simulink model "ScalarCalculator"  (R2021a)
settings: Solver=FixedStepDiscrete  StartTime=0.0  StopTime=10.0  RelTol=1e-3  EnableMultiTasking=on
libraries: simulink x2
settings Model: Creator=top one  LastModifiedBy=top one
settings DataIOCC: ReturnWorkspaceOutputs=off
settings OptimizationCC: DefaultParameterBehavior=Inlined  InlineInvariantSignals=on  EnableMemcpy=off  LifeSpan=1  EfficientTunableParamExpr=on
settings DebuggingCC: UnderspecifiedInitializationDetection=Classic  MergeDetectMultiDrivingBlocksExec=none  SFMachineParentedDataDiag=warning  ArithmeticOperatorsInVariantConditions=warning
settings ModelReferenceCC: PropagateSignalLabelsOutOfModel=off
settings SFSimCC: MATLABDynamicMemAlloc=off  CustomCodeUndefinedFunction=UseInterfaceOnly
settings RTWCC: SystemTargetFile=ert.tlc  GenCodeOnly=on  TemplateMakefile=ert_default_tmf  GenerateReport=on  IncludeHyperlinkInReport=on  LaunchReport=on  GenerateTraceInfo=on  GenerateTraceReport=on  GenerateTraceReportSl=on  GenerateTraceReportSf=on  GenerateTraceReportEml=on
settings CodeAppCC: ForceParamTrailComments=on  IgnoreCustomStorageClasses=off  OperatorAnnotations=on  SimulinkDataObjDesc=on  SFDataObjDesc=on  MATLABFcnDesc=on  InsertBlockDesc=on  StateflowObjectComments=on  MATLABSourceComments=on
settings ERTTargetCC: MultiwordLength=2048  GenerateSampleERTMain=on  InlinedParameterPlacement=NonHierarchical  ERTCustomFileTemplate=example_file_process.tlc

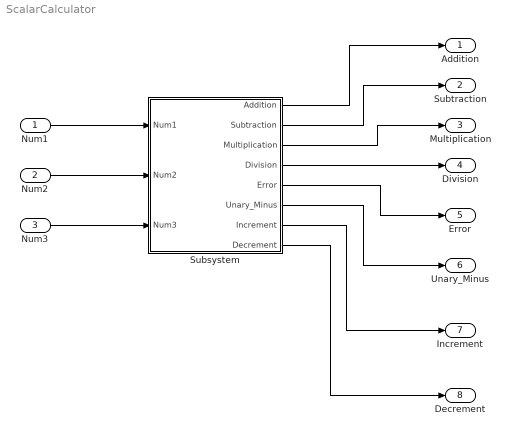
== system ScalarCalculator ==
  Num1 : Inport
  Num2 : Inport  Port=2
  Num3 : Inport  Port=3
  Subsystem : Subsystem
  Addition : Outport
  Subtraction : Outport  Port=2
  Multiplication : Outport  Port=3
  Division : Outport  Port=4
  Error : Outport  Port=5
  Unary_Minus : Outport  Port=6
  Increment : Outport  Port=7
  Decrement : Outport  Port=8
  wires:
  Subsystem/1(Addition) -> Addition/1
  Subsystem/2(Subtraction) -> Subtraction/1
  Subsystem/3(Multiplication) -> Multiplication/1
  Subsystem/4(Division) -> Division/1
  Subsystem/5(Error) -> Error/1
  Subsystem/6(Unary_Minus) -> Unary_Minus/1
  Subsystem/7(Increment) -> Increment/1
  Subsystem/8(Decrement) -> Decrement/1
  Num1/1 -> Subsystem/1(Num1)
  Num2/1 -> Subsystem/2(Num2)
  Num3/1 -> Subsystem/3(Num3)

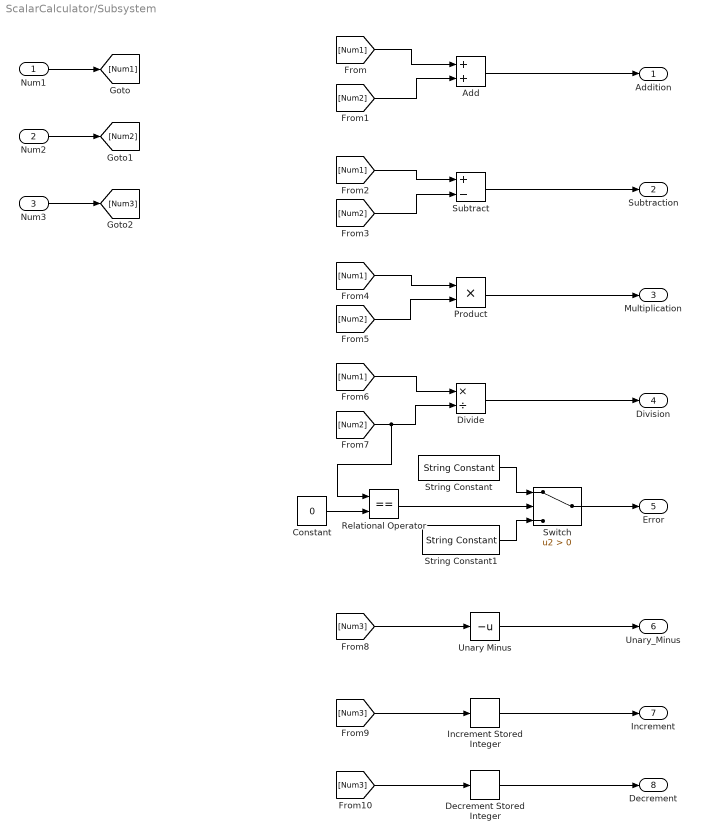
== system ScalarCalculator/Subsystem ==
  Num1 : Inport
  Num2 : Inport  Port=2
  Num3 : Inport  Port=3
  Add : Sum
  Constant : Constant  Value=0
  Decrement Stored Integer : simulink/Additional Math & Discrete/Additional Math: Increment - Decrement/Decrement Stored Integer
      settings: SourceProductBaseCode=SL
  Divide : Product  Inputs=*/
  Increment Stored Integer : simulink/Additional Math & Discrete/Additional Math: Increment - Decrement/Increment Stored Integer
  Product : Product
  Relational Operator : RelationalOperator  Operator===  OutDataTypeStr=boolean  RndMeth=Simplest
  String Constant : StringConstant  String="\"Error\""
  String Constant1 : StringConstant  String="\"No Error\""
  Subtract : Sum  Inputs=+-
  Switch : Switch  Criteria=u2 > Threshold
  Unary Minus : UnaryMinus
  Addition : Outport
  Subtraction : Outport  Port=2
  Multiplication : Outport  Port=3
  Division : Outport  Port=4
  Error : Outport  Port=5
  Unary_Minus : Outport  Port=6
  Increment : Outport  Port=7
  Decrement : Outport  Port=8
  wires:
  String Constant/1 -> Switch/1
  [Num2] -> Relational Operator/1, Divide/2
  [Num2] -> Add/2
  [Num3] -> Decrement Stored Integer/1
  [Num2] -> Subtract/2
  Relational Operator/1 -> Switch/2
  [Num1] -> Product/1
  [Num2] -> Product/2
  Constant/1 -> Relational Operator/2
  Switch/1 -> Error/1
  Divide/1 -> Division/1
  [Num3] -> Unary Minus/1
  [Num3] -> Increment Stored Integer/1
  Num1/1 -> [Num1]
  [Num1] -> Subtract/1
  Num2/1 -> [Num2]
  String Constant1/1 -> Switch/3
  [Num1] -> Add/1
  Num3/1 -> [Num3]
  Add/1 -> Addition/1
  Subtract/1 -> Subtraction/1
  [Num1] -> Divide/1
  Increment Stored Integer/1 -> Increment/1
  Product/1 -> Multiplication/1
  Unary Minus/1 -> Unary_Minus/1
  Decrement Stored Integer/1 -> Decrement/1
